simulink model "DFADAS2_SenFus_v1_201204RC_training_210115"  (R2018b)
settings: Solver=FixedStepDiscrete  StartTime=0.0  StopTime=inf  FixedStep=0.002  RelTol=1e-3  EnableMultiTasking=on
PreLoadFcn:
  | RTWConfigurationCB('preloadfcn', bdroot);
libraries: canmsglib x108, simulink x48, canfdmsglib x12
(part 18 of 28)

== system DFADAS2_SenFus_v1_201204RC_training_210115/Signal Input (Input)/Signal Input (50ms) (Input50)/Cmr/CmrInfo/R0 Information (R0Info)/CAN Diagnosis (CANDia)/RollingCounter Diagnosis (RllCntDia) ==
  note: RollingCounter Error Flag Discription:
      | 1 : Fault
      | 0 : Normal
  RllCntChk_ctRollingCounter : Inport
  Add : Sum  Inputs=+-
  Add1 : Sum  Inputs=+-
  Constant : Constant  OutDataTypeStr=single  SampleTime=-1
  Constant1 : Constant  Value=0  OutDataTypeStr=single  SampleTime=-1
  Constant2 : Constant  Value=-1  OutDataTypeStr=single  SampleTime=-1
  Constant3 : Constant  OutDataTypeStr=single  SampleTime=-1
  Data Type Conversion : DataTypeConversion  OutDataTypeStr=single
  Switch : Switch  Criteria=u2 ~= 0
  Switch1 : Switch  Threshold=14.5
  Unit Delay : UnitDelay  SampleTime=-1
  RllCntChk_efErrorFlag : Outport
  wires:
  Switch/1 -> RllCntChk_efErrorFlag/1
  Constant2/1 -> Switch1/1
  Switch1/1 -> Add/2
  Unit Delay/1 -> Switch1/3, Switch1/2
  Data Type Conversion/1 -> Unit Delay/1, Add/1
  Add1/1 -> Switch/2
  Constant3/1 -> Switch/1
  Constant1/1 -> Switch/3
  Constant/1 -> Add1/2
  Add/1 -> Add1/1
  RllCntChk_ctRollingCounter/1 -> Data Type Conversion/1

== system DFADAS2_SenFus_v1_201204RC_training_210115/Signal Input (Input)/Signal Input (50ms) (Input50)/Cmr/CmrInfo/R1 Information (R1Info)/CAN Diagnosis (CANDia)/Break State Diagnosis (BreStDia) ==
  note: Error Flag Discription:
      | 0 : Normal
      | 1 : Fault
  BreStDia_tiCANRxSmplT : Inport
  BreStDia_tiTLim : Inport  Port=2
  BreStDia_cfCANRxNewFlg : Inport  Port=3
  Add : Sum
  Add1 : Sum  Inputs=+-
  Constant : Constant  SampleTime=-1
  Constant1 : Constant  Value=0  SampleTime=-1
  Constant2 : Constant  Value=0  SampleTime=-1
  Constant3 : Constant  SampleTime=-1
  Divide : Product  Inputs=**
  Divide1 : Product  Inputs=/*
  Memory : Memory  InheritSampleTime=on
  Switch : Switch  Criteria=u2 ~= 0
  Switch1 : Switch
  BreStDia_efErrFlg : Outport
  wires:
  Constant1/1 -> Switch/1
  Constant/1 -> Switch/3
  Switch/1 -> Add/1, Divide/2
  Memory/1 -> Add/2
  Divide/1 -> Memory/1
  Add/1 -> Divide/1, Add1/2
  BreStDia_cfCANRxNewFlg/1 -> Switch/2
  BreStDia_tiCANRxSmplT/1 -> Divide1/1
  BreStDia_tiTLim/1 -> Divide1/2
  Add1/1 -> Switch1/2
  Constant2/1 -> Switch1/1
  Constant3/1 -> Switch1/3
  Switch1/1 -> BreStDia_efErrFlg/1
  Divide1/1 -> Add1/1

== system DFADAS2_SenFus_v1_201204RC_training_210115/Signal Input (Input)/Signal Input (50ms) (Input50)/Cmr/CmrInfo/R1 Information (R1Info)/CAN Diagnosis (CANDia)/CAN Frame DTC Generator (CANFrmDTCGtr) ==
  CANFrmDTCGtr_efBreStDiaErrFlg : Inport
  CANFrmDTCGtr_efChkSumDiaErrFlg : Inport  Port=2
  CANFrmDTCGtr_efRllCntDiaErrFlg : Inport  Port=3

== system DFADAS2_SenFus_v1_201204RC_training_210115/Signal Input (Input)/Signal Input (50ms) (Input50)/Cmr/CmrInfo/R1 Information (R1Info)/CAN Diagnosis (CANDia)/CheckSum Diagnosis (ChkSumDia) ==
  ChkSumDia_regCANMsgPrev : Inport
  Bit Check(BChk) : Subsystem  TreatAsAtomicUnit=on
      settings: RTWSystemCode=Nonreusable function
  CAN Message Data Extended (CMsgDaX) : S-Function  FunctionName=CANMsg_DataAcq  SFunctionDeploymentMode=off  EnableBusSupport=off  mask(CANMsg_DataExt){}
      mask help: This block extracts the raw data from the data field of the input CAN frame signal and outputs it as a 1-D array of data type uint8.
      mask Display:
      | color('blue');text(0.98,0.9,'NovSteeds','horizontalAlignment','right');color('black');text(0.5,0.5,'CAN Message\nData Extraction','horizontalAlignment','center');
      | port_label('input',1,'CAN_Msg');
      | port_label('output',1,'RawData');
  ChkSumDia_efErrFlg : Outport
  wires:
  Bit Check(BChk)/1(BChk_efErrFlg) -> ChkSumDia_efErrFlg/1
  ChkSumDia_regCANMsgPrev/1 -> CAN Message Data Extended (CMsgDaX)/1
  CAN Message Data Extended (CMsgDaX)/1 -> Bit Check(BChk)/1(BChk_bRawDa)

== system DFADAS2_SenFus_v1_201204RC_training_210115/Signal Input (Input)/Signal Input (50ms) (Input50)/Cmr/CmrInfo/R1 Information (R1Info)/CAN Diagnosis (CANDia)/RollingCounter Diagnosis (RllCntDia) ==
  note: RollingCounter Error Flag Discription:
      | 1 : Fault
      | 0 : Normal
  RllCntChk_ctRollingCounter : Inport
  Add : Sum  Inputs=+-
  Add1 : Sum  Inputs=+-
  Constant : Constant  OutDataTypeStr=single  SampleTime=-1
  Constant1 : Constant  Value=0  OutDataTypeStr=single  SampleTime=-1
  Constant2 : Constant  Value=-1  OutDataTypeStr=single  SampleTime=-1
  Constant3 : Constant  OutDataTypeStr=single  SampleTime=-1
  Data Type Conversion : DataTypeConversion  OutDataTypeStr=single
  Switch : Switch  Criteria=u2 ~= 0
  Switch1 : Switch  Threshold=14.5
  Unit Delay : UnitDelay  SampleTime=-1
  RllCntChk_efErrorFlag : Outport
  wires:
  RllCntChk_ctRollingCounter/1 -> Data Type Conversion/1
  Add/1 -> Add1/1
  Constant/1 -> Add1/2
  Constant1/1 -> Switch/3
  Constant3/1 -> Switch/1
  Add1/1 -> Switch/2
  Data Type Conversion/1 -> Add/1, Unit Delay/1
  Unit Delay/1 -> Switch1/2, Switch1/3
  Switch1/1 -> Add/2
  Constant2/1 -> Switch1/1
  Switch/1 -> RllCntChk_efErrorFlag/1

== system DFADAS2_SenFus_v1_201204RC_training_210115/Signal Input (Input)/Signal Input (50ms) (Input50)/Front Left Radar(S2) Objects Information (FLRdr)/S0 Data Frame Read/Enabled Subsystem/M0ObjInfo/If Action Subsystem1 ==
  msg : Inport
  "MValueSel " : Inport  Port=2
  obj_trufal : Inport  Port=3
  Action Port : ActionPort  ActionType=then
  Add : Sum
  Add2 : Sum
  MValueSel : Constant  Value=24
  MValueSel2 : Constant  Value=[1:24]
  Product : Product
  Scope1 : Scope
  Selector : Selector  InputPortWidth=240  IndexOptions=Index vector (port)  Indices=[1 3]  OutputSizes=1
  Selector1 : Selector  InputPortWidth=240  IndexOptions=Index vector (port)  Indices=[1 3]  OutputSizes=1
  M00ObjInfo : Outport
  M01ObjInfo : Outport  Port=2
  wires:
  Product/1 -> M01ObjInfo/1
  obj_trufal/1 -> Scope1/1, Product/2
  Selector1/1 -> Product/1
  Selector/1 -> M00ObjInfo/1
  "MValueSel "/1 -> Add2/1
  MValueSel2/1 -> Add2/2
  Add2/1 -> Add/1, Selector/2
  MValueSel/1 -> Add/2
  Add/1 -> Selector1/2
  msg/1 -> Selector1/1, Selector/1

== system DFADAS2_SenFus_v1_201204RC_training_210115/Signal Input (Input)/Signal Input (50ms) (Input50)/Front Left Radar(S2) Objects Information (FLRdr)/S0 Data Frame Read/Enabled Subsystem/M0ObjInfo/If Action Subsystem2 ==
  Action Port : ActionPort  ActionType=elseif
  Constant : Constant  Value=[0 0 0 0 0 0 0 0 0 0 0 0 0 0 0 0 0 0 0 0 0 0 0 0]
  Constant1 : Constant  Value=[0 0 0 0 0 0 0 0 0 0 0 0 0 0 0 0 0 0 0 0 0 0 0 0]
  ZeroObjInfo0 : Outport
  ZeroObjInfo1 : Outport  Port=2
  wires:
  Constant1/1 -> ZeroObjInfo1/1
  Constant/1 -> ZeroObjInfo0/1

== system DFADAS2_SenFus_v1_201204RC_training_210115/Signal Input (Input)/Signal Input (50ms) (Input50)/Front Left Radar(S2) Objects Information (FLRdr)/S0 Data Frame Read/Enabled Subsystem/M0ObjInfo/Subsystem1 ==
  const : Inport
  RemainderCnt : Inport  Port=2
  In : Inport  Port=3
  If : If  IfExpression=u1 >=0
  If Action Subsystem : Subsystem  TreatAsAtomicUnit=on
  If Action Subsystem1 : Subsystem  TreatAsAtomicUnit=on
  Merge : Merge
  Out : Outport
  wires:
  In/1 -> If Action Subsystem1/1(In1)
  const/1 -> If/1
  If/1 -> If Action Subsystem/Action
  If Action Subsystem1/1(Out1) -> Merge/2
  If/2 -> If Action Subsystem1/Action
  Merge/1 -> Out/1
  If Action Subsystem/1(Out1) -> Merge/1

== system DFADAS2_SenFus_v1_201204RC_training_210115/Signal Input (Input)/Signal Input (50ms) (Input50)/Front Left Radar(S2) Objects Information (FLRdr)/S0 Data Frame Read/Enabled Subsystem/M1ObjInfo1/If Action Subsystem1 ==
  msg : Inport
  "MValueSel " : Inport  Port=2
  "0bj_d4 " : Inport  Port=3
  Action Port : ActionPort  ActionType=then
  Add : Sum
  Add2 : Sum
  Gain : Gain  Gain=48
  MValueSel : Constant  Value=24
  MValueSel2 : Constant  Value=[1:24]
  Product : Product
  Scope3 : Scope
  Selector : Selector  InputPortWidth=240  IndexOptions=Index vector (port)  Indices=[1 3]  OutputSizes=1
  Selector1 : Selector  InputPortWidth=240  IndexOptions=Index vector (port)  Indices=[1 3]  OutputSizes=1
  M10ObjInfo : Outport
  M11ObjInfo : Outport  Port=2
  wires:
  Selector/1 -> M10ObjInfo/1
  Product/1 -> M11ObjInfo/1
  "0bj_d4 "/1 -> Scope3/1, Product/2
  "MValueSel "/1 -> Gain/1
  Gain/1 -> Add2/1
  msg/1 -> Selector1/1, Selector/1
  Add/1 -> Selector1/2
  MValueSel/1 -> Add/2
  Add2/1 -> Selector/2, Add/1
  MValueSel2/1 -> Add2/2
  Selector1/1 -> Product/1

== system DFADAS2_SenFus_v1_201204RC_training_210115/Signal Input (Input)/Signal Input (50ms) (Input50)/Front Left Radar(S2) Objects Information (FLRdr)/S0 Data Frame Read/Enabled Subsystem/M1ObjInfo1/If Action Subsystem2 ==
  Action Port : ActionPort  ActionType=elseif
  Constant : Constant  Value=[0 0 0 0 0 0 0 0 0 0 0 0 0 0 0 0 0 0 0 0 0 0 0 0]
  Constant1 : Constant  Value=[0 0 0 0 0 0 0 0 0 0 0 0 0 0 0 0 0 0 0 0 0 0 0 0]
  ZeroObjInfo0 : Outport
  ZeroObjInfo1 : Outport  Port=2
  wires:
  Constant/1 -> ZeroObjInfo0/1
  Constant1/1 -> ZeroObjInfo1/1

== system DFADAS2_SenFus_v1_201204RC_training_210115/Signal Input (Input)/Signal Input (50ms) (Input50)/Front Left Radar(S2) Objects Information (FLRdr)/S0 Data Frame Read/Enabled Subsystem/M1ObjInfo1/Subsystem1 ==
  const : Inport
  RemainderCnt : Inport  Port=2
  In : Inport  Port=3
  If : If  IfExpression=u1 >=0
  If Action Subsystem : Subsystem  TreatAsAtomicUnit=on
  If Action Subsystem1 : Subsystem  TreatAsAtomicUnit=on
  Merge : Merge
  Out : Outport
  wires:
  In/1 -> If Action Subsystem1/1(In1)
  const/1 -> If/1
  If/1 -> If Action Subsystem/Action
  If Action Subsystem1/1(Out1) -> Merge/2
  If/2 -> If Action Subsystem1/Action
  Merge/1 -> Out/1
  If Action Subsystem/1(Out1) -> Merge/1

== system DFADAS2_SenFus_v1_201204RC_training_210115/Signal Input (Input)/Signal Input (50ms) (Input50)/Front Left Radar(S2) Objects Information (FLRdr)/S0 Data Frame Read/Enabled Subsystem/M2ObjInfo/If Action Subsystem1 ==
  msg : Inport
  "MValueSel " : Inport  Port=2
  "obj_count_trorfa " : Inport  Port=3
  Action Port : ActionPort  ActionType=then
  Add : Sum
  Add2 : Sum
  Gain : Gain  Gain=48
  MValueSel : Constant  Value=24
  MValueSel2 : Constant  Value=[1:24]
  Product : Product
  Scope3 : Scope
  Selector : Selector  InputPortWidth=240  IndexOptions=Index vector (port)  Indices=[1 3]  OutputSizes=1
  Selector1 : Selector  InputPortWidth=240  IndexOptions=Index vector (port)  Indices=[1 3]  OutputSizes=1
  M20ObjInfo : Outport
  M21ObjInfo : Outport  Port=2
  wires:
  Product/1 -> M21ObjInfo/1
  "obj_count_trorfa "/1 -> Scope3/1, Product/2
  Selector1/1 -> Product/1
  Selector/1 -> M20ObjInfo/1
  MValueSel2/1 -> Add2/2
  Add2/1 -> Add/1, Selector/2
  MValueSel/1 -> Add/2
  Add/1 -> Selector1/2
  msg/1 -> Selector/1, Selector1/1
  Gain/1 -> Add2/1
  "MValueSel "/1 -> Gain/1

== system DFADAS2_SenFus_v1_201204RC_training_210115/Signal Input (Input)/Signal Input (50ms) (Input50)/Front Left Radar(S2) Objects Information (FLRdr)/S0 Data Frame Read/Enabled Subsystem/M2ObjInfo/If Action Subsystem2 ==
  Action Port : ActionPort  ActionType=elseif
  Constant : Constant  Value=[0 0 0 0 0 0 0 0 0 0 0 0 0 0 0 0 0 0 0 0 0 0 0 0]
  Constant1 : Constant  Value=[0 0 0 0 0 0 0 0 0 0 0 0 0 0 0 0 0 0 0 0 0 0 0 0]
  ZeroObjInfo0 : Outport
  ZeroObjInfo1 : Outport  Port=2
  wires:
  Constant1/1 -> ZeroObjInfo1/1
  Constant/1 -> ZeroObjInfo0/1

== system DFADAS2_SenFus_v1_201204RC_training_210115/Signal Input (Input)/Signal Input (50ms) (Input50)/Front Left Radar(S2) Objects Information (FLRdr)/S0 Data Frame Read/Enabled Subsystem/M2ObjInfo/Subsystem1 ==
  const : Inport
  RemainderCnt : Inport  Port=2
  In : Inport  Port=3
  If : If  IfExpression=u1 >=0
  If Action Subsystem : Subsystem  TreatAsAtomicUnit=on
  If Action Subsystem1 : Subsystem  TreatAsAtomicUnit=on
  Merge : Merge
  Out : Outport
  wires:
  In/1 -> If Action Subsystem1/1(In1)
  const/1 -> If/1
  If/1 -> If Action Subsystem/Action
  If Action Subsystem1/1(Out1) -> Merge/2
  If/2 -> If Action Subsystem1/Action
  Merge/1 -> Out/1
  If Action Subsystem/1(Out1) -> Merge/1

== system DFADAS2_SenFus_v1_201204RC_training_210115/Signal Input (Input)/Signal Input (50ms) (Input50)/Front Left Radar(S2) Objects Information (FLRdr)/S0 Data Frame Read/Enabled Subsystem/M3ObjInfo/If Action Subsystem1 ==
  msg : Inport
  "MValueSel " : Inport  Port=2
  obj_num : Inport  Port=3
  Action Port : ActionPort  ActionType=then
  Add : Sum
  Add2 : Sum
  Gain : Gain  Gain=48
  MValueSel : Constant  Value=24
  MValueSel2 : Constant  Value=[1:24]
  Product : Product
  Scope3 : Scope
  Selector : Selector  InputPortWidth=240  IndexOptions=Index vector (port)  Indices=[1 3]  OutputSizes=1
  Selector1 : Selector  InputPortWidth=240  IndexOptions=Index vector (port)  Indices=[1 3]  OutputSizes=1
  M30ObjInfo : Outport
  M31ObjInfo : Outport  Port=2
  wires:
  Product/1 -> M31ObjInfo/1
  obj_num/1 -> Scope3/1, Product/2
  Selector1/1 -> Product/1
  "MValueSel "/1 -> Gain/1
  Gain/1 -> Add2/1
  msg/1 -> Selector1/1, Selector/1
  Add/1 -> Selector1/2
  MValueSel/1 -> Add/2
  Add2/1 -> Selector/2, Add/1
  MValueSel2/1 -> Add2/2
  Selector/1 -> M30ObjInfo/1

== system DFADAS2_SenFus_v1_201204RC_training_210115/Signal Input (Input)/Signal Input (50ms) (Input50)/Front Left Radar(S2) Objects Information (FLRdr)/S0 Data Frame Read/Enabled Subsystem/M3ObjInfo/If Action Subsystem2 ==
  Action Port : ActionPort  ActionType=elseif
  Constant : Constant  Value=[0 0 0 0 0 0 0 0 0 0 0 0 0 0 0 0 0 0 0 0 0 0 0 0]
  Constant1 : Constant  Value=[0 0 0 0 0 0 0 0 0 0 0 0 0 0 0 0 0 0 0 0 0 0 0 0]
  ZeroObjInfo0 : Outport
  ZeroObjInfo1 : Outport  Port=2
  wires:
  Constant/1 -> ZeroObjInfo0/1
  Constant1/1 -> ZeroObjInfo1/1

== system DFADAS2_SenFus_v1_201204RC_training_210115/Signal Input (Input)/Signal Input (50ms) (Input50)/Front Left Radar(S2) Objects Information (FLRdr)/S0 Data Frame Read/Enabled Subsystem/M3ObjInfo/Subsystem1 ==
  const : Inport
  RemainderCnt : Inport  Port=2
  In : Inport  Port=3
  If : If  IfExpression=u1 >=0
  If Action Subsystem : Subsystem  TreatAsAtomicUnit=on
  If Action Subsystem1 : Subsystem  TreatAsAtomicUnit=on
  Merge : Merge
  Out : Outport
  wires:
  In/1 -> If Action Subsystem1/1(In1)
  const/1 -> If/1
  If/1 -> If Action Subsystem/Action
  If Action Subsystem1/1(Out1) -> Merge/2
  If/2 -> If Action Subsystem1/Action
  Merge/1 -> Out/1
  If Action Subsystem/1(Out1) -> Merge/1

== system DFADAS2_SenFus_v1_201204RC_training_210115/Signal Input (Input)/Signal Input (50ms) (Input50)/Front Left Radar(S2) Objects Information (FLRdr)/S0 Data Frame Read/Enabled Subsystem/M4ObjInfo1/If Action Subsystem1 ==
  msg : Inport
  "MValueSel " : Inport  Port=2
  "obj_num " : Inport  Port=3
  Action Port : ActionPort  ActionType=then
  Add : Sum
  Add2 : Sum
  Gain : Gain  Gain=48
  MValueSel : Constant  Value=24
  MValueSel2 : Constant  Value=[1:24]
  Product : Product
  Scope3 : Scope
  Selector : Selector  InputPortWidth=240  IndexOptions=Index vector (port)  Indices=[1 3]  OutputSizes=1
  Selector1 : Selector  InputPortWidth=240  IndexOptions=Index vector (port)  Indices=[1 3]  OutputSizes=1
  M40ObjInfo : Outport
  M41ObjInfo : Outport  Port=2
  wires:
  Product/1 -> M41ObjInfo/1
  "obj_num "/1 -> Scope3/1, Product/2
  Selector1/1 -> Product/1
  Selector/1 -> M40ObjInfo/1
  MValueSel2/1 -> Add2/2
  Add2/1 -> Add/1, Selector/2
  MValueSel/1 -> Add/2
  Add/1 -> Selector1/2
  msg/1 -> Selector/1, Selector1/1
  Gain/1 -> Add2/1
  "MValueSel "/1 -> Gain/1

== system DFADAS2_SenFus_v1_201204RC_training_210115/Signal Input (Input)/Signal Input (50ms) (Input50)/Front Left Radar(S2) Objects Information (FLRdr)/S0 Data Frame Read/Enabled Subsystem/M4ObjInfo1/If Action Subsystem2 ==
  Action Port : ActionPort  ActionType=elseif
  Constant : Constant  Value=[0 0 0 0 0 0 0 0 0 0 0 0 0 0 0 0 0 0 0 0 0 0 0 0]
  Constant1 : Constant  Value=[0 0 0 0 0 0 0 0 0 0 0 0 0 0 0 0 0 0 0 0 0 0 0 0]
  ZeroObjInfo0 : Outport
  ZeroObjInfo1 : Outport  Port=2
  wires:
  Constant1/1 -> ZeroObjInfo1/1
  Constant/1 -> ZeroObjInfo0/1

== system DFADAS2_SenFus_v1_201204RC_training_210115/Signal Input (Input)/Signal Input (50ms) (Input50)/Front Left Radar(S2) Objects Information (FLRdr)/S0 Data Frame Read/Enabled Subsystem/M4ObjInfo1/Subsystem1 ==
  const : Inport
  RemainderCnt : Inport  Port=2
  In : Inport  Port=3
  If : If  IfExpression=u1 >=0
  If Action Subsystem : Subsystem  TreatAsAtomicUnit=on
  If Action Subsystem1 : Subsystem  TreatAsAtomicUnit=on
  Merge : Merge
  Out : Outport
  wires:
  In/1 -> If Action Subsystem1/1(In1)
  const/1 -> If/1
  If/1 -> If Action Subsystem/Action
  If Action Subsystem1/1(Out1) -> Merge/2
  If/2 -> If Action Subsystem1/Action
  Merge/1 -> Out/1
  If Action Subsystem/1(Out1) -> Merge/1

== system DFADAS2_SenFus_v1_201204RC_training_210115/Signal Input (Input)/Signal Input (50ms) (Input50)/Front Left Radar(S2) Objects Information (FLRdr)/S0 Data Frame Read/Enabled Subsystem/Unpack/If Action Subsystem ==
  msg : Inport
  Action Port : ActionPort  ActionType=then
  Unpack : Subsystem
  FLRdrObjInfo : Outport
  MValue : Outport  Port=2
  wires:
  Unpack/2(MValue) -> MValue/1
  msg/1 -> Unpack/1(msg)
  Unpack/1(FLRdrObjInfo) -> FLRdrObjInfo/1

== system DFADAS2_SenFus_v1_201204RC_training_210115/Signal Input (Input)/Signal Input (50ms) (Input50)/Front Left Radar(S2) Objects Information (FLRdr)/S0 Data Frame Read/Enabled Subsystem/Unpack/If Action Subsystem1 ==
  Action Port : ActionPort  ActionType=elseif
  Constant : Constant  Value=99
  DflMValue : Outport
  wires:
  Constant/1 -> DflMValue/1

== system DFADAS2_SenFus_v1_201204RC_training_210115/Signal Input (Input)/Signal Input (50ms) (Input50)/Front Right Radar(S3) Objects Information (FRRdr)/S0 Data Frame Read/Enabled Subsystem/M0ObjInfo/If Action Subsystem1 ==
  msg : Inport
  "MValueSel " : Inport  Port=2
  obj_trufal : Inport  Port=3
  Action Port : ActionPort  ActionType=then
  Add : Sum
  Add2 : Sum
  MValueSel : Constant  Value=24
  MValueSel2 : Constant  Value=[1:24]
  Product : Product
  Scope1 : Scope
  Selector : Selector  InputPortWidth=240  IndexOptions=Index vector (port)  Indices=[1 3]  OutputSizes=1
  Selector1 : Selector  InputPortWidth=240  IndexOptions=Index vector (port)  Indices=[1 3]  OutputSizes=1
  M00ObjInfo : Outport
  M01ObjInfo : Outport  Port=2
  wires:
  msg/1 -> Selector/1, Selector1/1
  Add/1 -> Selector1/2
  MValueSel/1 -> Add/2
  Add2/1 -> Selector/2, Add/1
  MValueSel2/1 -> Add2/2
  "MValueSel "/1 -> Add2/1
  Selector/1 -> M00ObjInfo/1
  Selector1/1 -> Product/1
  obj_trufal/1 -> Product/2, Scope1/1
  Product/1 -> M01ObjInfo/1

== system DFADAS2_SenFus_v1_201204RC_training_210115/Signal Input (Input)/Signal Input (50ms) (Input50)/Front Right Radar(S3) Objects Information (FRRdr)/S0 Data Frame Read/Enabled Subsystem/M0ObjInfo/If Action Subsystem2 ==
  Action Port : ActionPort  ActionType=elseif
  Constant : Constant  Value=[0 0 0 0 0 0 0 0 0 0 0 0 0 0 0 0 0 0 0 0 0 0 0 0]
  Constant1 : Constant  Value=[0 0 0 0 0 0 0 0 0 0 0 0 0 0 0 0 0 0 0 0 0 0 0 0]
  ZeroObjInfo0 : Outport
  ZeroObjInfo1 : Outport  Port=2
  wires:
  Constant/1 -> ZeroObjInfo0/1
  Constant1/1 -> ZeroObjInfo1/1

== system DFADAS2_SenFus_v1_201204RC_training_210115/Signal Input (Input)/Signal Input (50ms) (Input50)/Front Right Radar(S3) Objects Information (FRRdr)/S0 Data Frame Read/Enabled Subsystem/M0ObjInfo/Subsystem1 ==
  const : Inport
  RemainderCnt : Inport  Port=2
  In : Inport  Port=3
  If : If  IfExpression=u1 >=0
  If Action Subsystem : Subsystem  TreatAsAtomicUnit=on
  If Action Subsystem1 : Subsystem  TreatAsAtomicUnit=on
  Merge : Merge
  Out : Outport
  wires:
  If Action Subsystem/1(Out1) -> Merge/1
  Merge/1 -> Out/1
  If/2 -> If Action Subsystem1/Action
  If Action Subsystem1/1(Out1) -> Merge/2
  If/1 -> If Action Subsystem/Action
  const/1 -> If/1
  In/1 -> If Action Subsystem1/1(In1)

== system DFADAS2_SenFus_v1_201204RC_training_210115/Signal Input (Input)/Signal Input (50ms) (Input50)/Front Right Radar(S3) Objects Information (FRRdr)/S0 Data Frame Read/Enabled Subsystem/M1ObjInfo1/If Action Subsystem1 ==
  msg : Inport
  "MValueSel " : Inport  Port=2
  "0bj_d4 " : Inport  Port=3
  Action Port : ActionPort  ActionType=then
  Add : Sum
  Add2 : Sum
  Gain : Gain  Gain=48
  MValueSel : Constant  Value=24
  MValueSel2 : Constant  Value=[1:24]
  Product : Product
  Scope3 : Scope
  Selector : Selector  InputPortWidth=240  IndexOptions=Index vector (port)  Indices=[1 3]  OutputSizes=1
  Selector1 : Selector  InputPortWidth=240  IndexOptions=Index vector (port)  Indices=[1 3]  OutputSizes=1
  M10ObjInfo : Outport
  M11ObjInfo : Outport  Port=2
  wires:
  Selector1/1 -> Product/1
  MValueSel2/1 -> Add2/2
  Add2/1 -> Add/1, Selector/2
  MValueSel/1 -> Add/2
  Add/1 -> Selector1/2
  msg/1 -> Selector/1, Selector1/1
  Gain/1 -> Add2/1
  "MValueSel "/1 -> Gain/1
  "0bj_d4 "/1 -> Product/2, Scope3/1
  Product/1 -> M11ObjInfo/1
  Selector/1 -> M10ObjInfo/1

== system DFADAS2_SenFus_v1_201204RC_training_210115/Signal Input (Input)/Signal Input (50ms) (Input50)/Front Right Radar(S3) Objects Information (FRRdr)/S0 Data Frame Read/Enabled Subsystem/M1ObjInfo1/If Action Subsystem2 ==
  Action Port : ActionPort  ActionType=elseif
  Constant : Constant  Value=[0 0 0 0 0 0 0 0 0 0 0 0 0 0 0 0 0 0 0 0 0 0 0 0]
  Constant1 : Constant  Value=[0 0 0 0 0 0 0 0 0 0 0 0 0 0 0 0 0 0 0 0 0 0 0 0]
  ZeroObjInfo0 : Outport
  ZeroObjInfo1 : Outport  Port=2
  wires:
  Constant1/1 -> ZeroObjInfo1/1
  Constant/1 -> ZeroObjInfo0/1

== system DFADAS2_SenFus_v1_201204RC_training_210115/Signal Input (Input)/Signal Input (50ms) (Input50)/Front Right Radar(S3) Objects Information (FRRdr)/S0 Data Frame Read/Enabled Subsystem/M1ObjInfo1/Subsystem1 ==
  const : Inport
  RemainderCnt : Inport  Port=2
  In : Inport  Port=3
  If : If  IfExpression=u1 >=0
  If Action Subsystem : Subsystem  TreatAsAtomicUnit=on
  If Action Subsystem1 : Subsystem  TreatAsAtomicUnit=on
  Merge : Merge
  Out : Outport
  wires:
  If Action Subsystem/1(Out1) -> Merge/1
  Merge/1 -> Out/1
  If/2 -> If Action Subsystem1/Action
  If Action Subsystem1/1(Out1) -> Merge/2
  If/1 -> If Action Subsystem/Action
  const/1 -> If/1
  In/1 -> If Action Subsystem1/1(In1)

== system DFADAS2_SenFus_v1_201204RC_training_210115/Signal Input (Input)/Signal Input (50ms) (Input50)/Front Right Radar(S3) Objects Information (FRRdr)/S0 Data Frame Read/Enabled Subsystem/M2ObjInfo/If Action Subsystem1 ==
  msg : Inport
  "MValueSel " : Inport  Port=2
  "obj_count_trorfa " : Inport  Port=3
  Action Port : ActionPort  ActionType=then
  Add : Sum
  Add2 : Sum
  Gain : Gain  Gain=48
  MValueSel : Constant  Value=24
  MValueSel2 : Constant  Value=[1:24]
  Product : Product
  Scope3 : Scope
  Selector : Selector  InputPortWidth=240  IndexOptions=Index vector (port)  Indices=[1 3]  OutputSizes=1
  Selector1 : Selector  InputPortWidth=240  IndexOptions=Index vector (port)  Indices=[1 3]  OutputSizes=1
  M20ObjInfo : Outport
  M21ObjInfo : Outport  Port=2
  wires:
  "MValueSel "/1 -> Gain/1
  Gain/1 -> Add2/1
  msg/1 -> Selector1/1, Selector/1
  Add/1 -> Selector1/2
  MValueSel/1 -> Add/2
  Add2/1 -> Selector/2, Add/1
  MValueSel2/1 -> Add2/2
  Selector/1 -> M20ObjInfo/1
  Selector1/1 -> Product/1
  "obj_count_trorfa "/1 -> Product/2, Scope3/1
  Product/1 -> M21ObjInfo/1

== system DFADAS2_SenFus_v1_201204RC_training_210115/Signal Input (Input)/Signal Input (50ms) (Input50)/Front Right Radar(S3) Objects Information (FRRdr)/S0 Data Frame Read/Enabled Subsystem/M2ObjInfo/If Action Subsystem2 ==
  Action Port : ActionPort  ActionType=elseif
  Constant : Constant  Value=[0 0 0 0 0 0 0 0 0 0 0 0 0 0 0 0 0 0 0 0 0 0 0 0]
  Constant1 : Constant  Value=[0 0 0 0 0 0 0 0 0 0 0 0 0 0 0 0 0 0 0 0 0 0 0 0]
  ZeroObjInfo0 : Outport
  ZeroObjInfo1 : Outport  Port=2
  wires:
  Constant/1 -> ZeroObjInfo0/1
  Constant1/1 -> ZeroObjInfo1/1

== system DFADAS2_SenFus_v1_201204RC_training_210115/Signal Input (Input)/Signal Input (50ms) (Input50)/Front Right Radar(S3) Objects Information (FRRdr)/S0 Data Frame Read/Enabled Subsystem/M2ObjInfo/Subsystem1 ==
  const : Inport
  RemainderCnt : Inport  Port=2
  In : Inport  Port=3
  If : If  IfExpression=u1 >=0
  If Action Subsystem : Subsystem  TreatAsAtomicUnit=on
  If Action Subsystem1 : Subsystem  TreatAsAtomicUnit=on
  Merge : Merge
  Out : Outport
  wires:
  If Action Subsystem/1(Out1) -> Merge/1
  Merge/1 -> Out/1
  If/2 -> If Action Subsystem1/Action
  If Action Subsystem1/1(Out1) -> Merge/2
  If/1 -> If Action Subsystem/Action
  const/1 -> If/1
  In/1 -> If Action Subsystem1/1(In1)

== system DFADAS2_SenFus_v1_201204RC_training_210115/Signal Input (Input)/Signal Input (50ms) (Input50)/Front Right Radar(S3) Objects Information (FRRdr)/S0 Data Frame Read/Enabled Subsystem/M3ObjInfo/If Action Subsystem1 ==
  msg : Inport
  "MValueSel " : Inport  Port=2
  obj_num : Inport  Port=3
  Action Port : ActionPort  ActionType=then
  Add : Sum
  Add2 : Sum
  Gain : Gain  Gain=48
  MValueSel : Constant  Value=24
  MValueSel2 : Constant  Value=[1:24]
  Product : Product
  Scope3 : Scope
  Selector : Selector  InputPortWidth=240  IndexOptions=Index vector (port)  Indices=[1 3]  OutputSizes=1
  Selector1 : Selector  InputPortWidth=240  IndexOptions=Index vector (port)  Indices=[1 3]  OutputSizes=1
  M30ObjInfo : Outport
  M31ObjInfo : Outport  Port=2
  wires:
  Selector/1 -> M30ObjInfo/1
  MValueSel2/1 -> Add2/2
  Add2/1 -> Add/1, Selector/2
  MValueSel/1 -> Add/2
  Add/1 -> Selector1/2
  msg/1 -> Selector/1, Selector1/1
  Gain/1 -> Add2/1
  "MValueSel "/1 -> Gain/1
  Selector1/1 -> Product/1
  obj_num/1 -> Product/2, Scope3/1
  Product/1 -> M31ObjInfo/1

== system DFADAS2_SenFus_v1_201204RC_training_210115/Signal Input (Input)/Signal Input (50ms) (Input50)/Front Right Radar(S3) Objects Information (FRRdr)/S0 Data Frame Read/Enabled Subsystem/M3ObjInfo/If Action Subsystem2 ==
  Action Port : ActionPort  ActionType=elseif
  Constant : Constant  Value=[0 0 0 0 0 0 0 0 0 0 0 0 0 0 0 0 0 0 0 0 0 0 0 0]
  Constant1 : Constant  Value=[0 0 0 0 0 0 0 0 0 0 0 0 0 0 0 0 0 0 0 0 0 0 0 0]
  ZeroObjInfo0 : Outport
  ZeroObjInfo1 : Outport  Port=2
  wires:
  Constant1/1 -> ZeroObjInfo1/1
  Constant/1 -> ZeroObjInfo0/1

== system DFADAS2_SenFus_v1_201204RC_training_210115/Signal Input (Input)/Signal Input (50ms) (Input50)/Front Right Radar(S3) Objects Information (FRRdr)/S0 Data Frame Read/Enabled Subsystem/M3ObjInfo/Subsystem1 ==
  const : Inport
  RemainderCnt : Inport  Port=2
  In : Inport  Port=3
  If : If  IfExpression=u1 >=0
  If Action Subsystem : Subsystem  TreatAsAtomicUnit=on
  If Action Subsystem1 : Subsystem  TreatAsAtomicUnit=on
  Merge : Merge
  Out : Outport
  wires:
  If Action Subsystem/1(Out1) -> Merge/1
  Merge/1 -> Out/1
  If/2 -> If Action Subsystem1/Action
  If Action Subsystem1/1(Out1) -> Merge/2
  If/1 -> If Action Subsystem/Action
  const/1 -> If/1
  In/1 -> If Action Subsystem1/1(In1)

== system DFADAS2_SenFus_v1_201204RC_training_210115/Signal Input (Input)/Signal Input (50ms) (Input50)/Front Right Radar(S3) Objects Information (FRRdr)/S0 Data Frame Read/Enabled Subsystem/M4ObjInfo1/If Action Subsystem1 ==
  msg : Inport
  "MValueSel " : Inport  Port=2
  "obj_num " : Inport  Port=3
  Action Port : ActionPort  ActionType=then
  Add : Sum
  Add2 : Sum
  Gain : Gain  Gain=48
  MValueSel : Constant  Value=24
  MValueSel2 : Constant  Value=[1:24]
  Product : Product
  Scope3 : Scope
  Selector : Selector  InputPortWidth=240  IndexOptions=Index vector (port)  Indices=[1 3]  OutputSizes=1
  Selector1 : Selector  InputPortWidth=240  IndexOptions=Index vector (port)  Indices=[1 3]  OutputSizes=1
  M40ObjInfo : Outport
  M41ObjInfo : Outport  Port=2
  wires:
  "MValueSel "/1 -> Gain/1
  Gain/1 -> Add2/1
  msg/1 -> Selector1/1, Selector/1
  Add/1 -> Selector1/2
  MValueSel/1 -> Add/2
  Add2/1 -> Selector/2, Add/1
  MValueSel2/1 -> Add2/2
  Selector/1 -> M40ObjInfo/1
  Selector1/1 -> Product/1
  "obj_num "/1 -> Product/2, Scope3/1
  Product/1 -> M41ObjInfo/1

== system DFADAS2_SenFus_v1_201204RC_training_210115/Signal Input (Input)/Signal Input (50ms) (Input50)/Front Right Radar(S3) Objects Information (FRRdr)/S0 Data Frame Read/Enabled Subsystem/M4ObjInfo1/If Action Subsystem2 ==
  Action Port : ActionPort  ActionType=elseif
  Constant : Constant  Value=[0 0 0 0 0 0 0 0 0 0 0 0 0 0 0 0 0 0 0 0 0 0 0 0]
  Constant1 : Constant  Value=[0 0 0 0 0 0 0 0 0 0 0 0 0 0 0 0 0 0 0 0 0 0 0 0]
  ZeroObjInfo0 : Outport
  ZeroObjInfo1 : Outport  Port=2
  wires:
  Constant/1 -> ZeroObjInfo0/1
  Constant1/1 -> ZeroObjInfo1/1

== system DFADAS2_SenFus_v1_201204RC_training_210115/Signal Input (Input)/Signal Input (50ms) (Input50)/Front Right Radar(S3) Objects Information (FRRdr)/S0 Data Frame Read/Enabled Subsystem/M4ObjInfo1/Subsystem1 ==
  const : Inport
  RemainderCnt : Inport  Port=2
  In : Inport  Port=3
  If : If  IfExpression=u1 >=0
  If Action Subsystem : Subsystem  TreatAsAtomicUnit=on
  If Action Subsystem1 : Subsystem  TreatAsAtomicUnit=on
  Merge : Merge
  Out : Outport
  wires:
  If Action Subsystem/1(Out1) -> Merge/1
  Merge/1 -> Out/1
  If/2 -> If Action Subsystem1/Action
  If Action Subsystem1/1(Out1) -> Merge/2
  If/1 -> If Action Subsystem/Action
  const/1 -> If/1
  In/1 -> If Action Subsystem1/1(In1)

== system DFADAS2_SenFus_v1_201204RC_training_210115/Signal Input (Input)/Signal Input (50ms) (Input50)/Front Right Radar(S3) Objects Information (FRRdr)/S0 Data Frame Read/Enabled Subsystem/Unpack/If Action Subsystem ==
  msg : Inport
  Action Port : ActionPort  ActionType=then
  Unpack : Subsystem
  FRRdrObjInfo : Outport
  MValue : Outport  Port=2
  wires:
  Unpack/2(MValue) -> MValue/1
  msg/1 -> Unpack/1(msg)
  Unpack/1(FRRdrObjInfo) -> FRRdrObjInfo/1

== system DFADAS2_SenFus_v1_201204RC_training_210115/Signal Input (Input)/Signal Input (50ms) (Input50)/Front Right Radar(S3) Objects Information (FRRdr)/S0 Data Frame Read/Enabled Subsystem/Unpack/If Action Subsystem1 ==
  Action Port : ActionPort  ActionType=elseif
  Constant : Constant  Value=99
  DflMValue : Outport
  wires:
  Constant/1 -> DflMValue/1

== system DFADAS2_SenFus_v1_201204RC_training_210115/Signal Input (Input)/Signal Input (50ms) (Input50)/Rear Left Radar(S0) Objects Information (RLRdr)/S0 Data Frame Read/Enabled Subsystem/M0ObjInfo/If Action Subsystem1 ==
  msg : Inport
  "MValueSel " : Inport  Port=2
  obj_trufal : Inport  Port=3
  Action Port : ActionPort  ActionType=then
  Add : Sum
  Add2 : Sum
  MValueSel : Constant  Value=24
  MValueSel2 : Constant  Value=[1:24]
  Product : Product
  Scope1 : Scope
  Selector : Selector  InputPortWidth=240  IndexOptions=Index vector (port)  Indices=[1 3]  OutputSizes=1
  Selector1 : Selector  InputPortWidth=240  IndexOptions=Index vector (port)  Indices=[1 3]  OutputSizes=1
  M00ObjInfo : Outport
  M01ObjInfo : Outport  Port=2
  wires:
  msg/1 -> Selector/1, Selector1/1
  Add/1 -> Selector1/2
  MValueSel/1 -> Add/2
  Add2/1 -> Selector/2, Add/1
  MValueSel2/1 -> Add2/2
  "MValueSel "/1 -> Add2/1
  Selector/1 -> M00ObjInfo/1
  Selector1/1 -> Product/1
  obj_trufal/1 -> Product/2, Scope1/1
  Product/1 -> M01ObjInfo/1

== system DFADAS2_SenFus_v1_201204RC_training_210115/Signal Input (Input)/Signal Input (50ms) (Input50)/Rear Left Radar(S0) Objects Information (RLRdr)/S0 Data Frame Read/Enabled Subsystem/M0ObjInfo/If Action Subsystem2 ==
  Action Port : ActionPort  ActionType=elseif
  Constant : Constant  Value=[0 0 0 0 0 0 0 0 0 0 0 0 0 0 0 0 0 0 0 0 0 0 0 0]
  Constant1 : Constant  Value=[0 0 0 0 0 0 0 0 0 0 0 0 0 0 0 0 0 0 0 0 0 0 0 0]
  ZeroObjInfo0 : Outport
  ZeroObjInfo1 : Outport  Port=2
  wires:
  Constant/1 -> ZeroObjInfo0/1
  Constant1/1 -> ZeroObjInfo1/1

== system DFADAS2_SenFus_v1_201204RC_training_210115/Signal Input (Input)/Signal Input (50ms) (Input50)/Rear Left Radar(S0) Objects Information (RLRdr)/S0 Data Frame Read/Enabled Subsystem/M0ObjInfo/Subsystem1 ==
  const : Inport
  RemainderCnt : Inport  Port=2
  In : Inport  Port=3
  If : If  IfExpression=u1 >=0
  If Action Subsystem : Subsystem  TreatAsAtomicUnit=on
  If Action Subsystem1 : Subsystem  TreatAsAtomicUnit=on
  Merge : Merge
  Out : Outport
  wires:
  If Action Subsystem/1(Out1) -> Merge/1
  Merge/1 -> Out/1
  If/2 -> If Action Subsystem1/Action
  If Action Subsystem1/1(Out1) -> Merge/2
  If/1 -> If Action Subsystem/Action
  const/1 -> If/1
  In/1 -> If Action Subsystem1/1(In1)

== system DFADAS2_SenFus_v1_201204RC_training_210115/Signal Input (Input)/Signal Input (50ms) (Input50)/Rear Left Radar(S0) Objects Information (RLRdr)/S0 Data Frame Read/Enabled Subsystem/M1ObjInfo1/If Action Subsystem1 ==
  msg : Inport
  "MValueSel " : Inport  Port=2
  "0bj_d4 " : Inport  Port=3
  Action Port : ActionPort  ActionType=then
  Add : Sum
  Add2 : Sum
  Gain : Gain  Gain=48
  MValueSel : Constant  Value=24
  MValueSel2 : Constant  Value=[1:24]
  Product : Product
  Scope3 : Scope
  Selector : Selector  InputPortWidth=240  IndexOptions=Index vector (port)  Indices=[1 3]  OutputSizes=1
  Selector1 : Selector  InputPortWidth=240  IndexOptions=Index vector (port)  Indices=[1 3]  OutputSizes=1
  M10ObjInfo : Outport
  M11ObjInfo : Outport  Port=2
  wires:
  Selector1/1 -> Product/1
  MValueSel2/1 -> Add2/2
  Add2/1 -> Add/1, Selector/2
  MValueSel/1 -> Add/2
  Add/1 -> Selector1/2
  msg/1 -> Selector/1, Selector1/1
  Gain/1 -> Add2/1
  "MValueSel "/1 -> Gain/1
  "0bj_d4 "/1 -> Product/2, Scope3/1
  Product/1 -> M11ObjInfo/1
  Selector/1 -> M10ObjInfo/1

== system DFADAS2_SenFus_v1_201204RC_training_210115/Signal Input (Input)/Signal Input (50ms) (Input50)/Rear Left Radar(S0) Objects Information (RLRdr)/S0 Data Frame Read/Enabled Subsystem/M1ObjInfo1/If Action Subsystem2 ==
  Action Port : ActionPort  ActionType=elseif
  Constant : Constant  Value=[0 0 0 0 0 0 0 0 0 0 0 0 0 0 0 0 0 0 0 0 0 0 0 0]
  Constant1 : Constant  Value=[0 0 0 0 0 0 0 0 0 0 0 0 0 0 0 0 0 0 0 0 0 0 0 0]
  ZeroObjInfo0 : Outport
  ZeroObjInfo1 : Outport  Port=2
  wires:
  Constant1/1 -> ZeroObjInfo1/1
  Constant/1 -> ZeroObjInfo0/1

== system DFADAS2_SenFus_v1_201204RC_training_210115/Signal Input (Input)/Signal Input (50ms) (Input50)/Rear Left Radar(S0) Objects Information (RLRdr)/S0 Data Frame Read/Enabled Subsystem/M1ObjInfo1/Subsystem1 ==
  const : Inport
  RemainderCnt : Inport  Port=2
  In : Inport  Port=3
  If : If  IfExpression=u1 >=0
  If Action Subsystem : Subsystem  TreatAsAtomicUnit=on
  If Action Subsystem1 : Subsystem  TreatAsAtomicUnit=on
  Merge : Merge
  Out : Outport
  wires:
  If Action Subsystem/1(Out1) -> Merge/1
  Merge/1 -> Out/1
  If/2 -> If Action Subsystem1/Action
  If Action Subsystem1/1(Out1) -> Merge/2
  If/1 -> If Action Subsystem/Action
  const/1 -> If/1
  In/1 -> If Action Subsystem1/1(In1)

== system DFADAS2_SenFus_v1_201204RC_training_210115/Signal Input (Input)/Signal Input (50ms) (Input50)/Rear Left Radar(S0) Objects Information (RLRdr)/S0 Data Frame Read/Enabled Subsystem/M2ObjInfo/If Action Subsystem1 ==
  msg : Inport
  "MValueSel " : Inport  Port=2
  "obj_count_trorfa " : Inport  Port=3
  Action Port : ActionPort  ActionType=then
  Add : Sum
  Add2 : Sum
  Gain : Gain  Gain=48
  MValueSel : Constant  Value=24
  MValueSel2 : Constant  Value=[1:24]
  Product : Product
  Scope3 : Scope
  Selector : Selector  InputPortWidth=240  IndexOptions=Index vector (port)  Indices=[1 3]  OutputSizes=1
  Selector1 : Selector  InputPortWidth=240  IndexOptions=Index vector (port)  Indices=[1 3]  OutputSizes=1
  M20ObjInfo : Outport
  M21ObjInfo : Outport  Port=2
  wires:
  "MValueSel "/1 -> Gain/1
  Gain/1 -> Add2/1
  msg/1 -> Selector1/1, Selector/1
  Add/1 -> Selector1/2
  MValueSel/1 -> Add/2
  Add2/1 -> Selector/2, Add/1
  MValueSel2/1 -> Add2/2
  Selector/1 -> M20ObjInfo/1
  Selector1/1 -> Product/1
  "obj_count_trorfa "/1 -> Product/2, Scope3/1
  Product/1 -> M21ObjInfo/1

== system DFADAS2_SenFus_v1_201204RC_training_210115/Signal Input (Input)/Signal Input (50ms) (Input50)/Rear Left Radar(S0) Objects Information (RLRdr)/S0 Data Frame Read/Enabled Subsystem/M2ObjInfo/If Action Subsystem2 ==
  Action Port : ActionPort  ActionType=elseif
  Constant : Constant  Value=[0 0 0 0 0 0 0 0 0 0 0 0 0 0 0 0 0 0 0 0 0 0 0 0]
  Constant1 : Constant  Value=[0 0 0 0 0 0 0 0 0 0 0 0 0 0 0 0 0 0 0 0 0 0 0 0]
  ZeroObjInfo0 : Outport
  ZeroObjInfo1 : Outport  Port=2
  wires:
  Constant/1 -> ZeroObjInfo0/1
  Constant1/1 -> ZeroObjInfo1/1

== system DFADAS2_SenFus_v1_201204RC_training_210115/Signal Input (Input)/Signal Input (50ms) (Input50)/Rear Left Radar(S0) Objects Information (RLRdr)/S0 Data Frame Read/Enabled Subsystem/M2ObjInfo/Subsystem1 ==
  const : Inport
  RemainderCnt : Inport  Port=2
  In : Inport  Port=3
  If : If  IfExpression=u1 >=0
  If Action Subsystem : Subsystem  TreatAsAtomicUnit=on
  If Action Subsystem1 : Subsystem  TreatAsAtomicUnit=on
  Merge : Merge
  Out : Outport
  wires:
  If Action Subsystem/1(Out1) -> Merge/1
  Merge/1 -> Out/1
  If/2 -> If Action Subsystem1/Action
  If Action Subsystem1/1(Out1) -> Merge/2
  If/1 -> If Action Subsystem/Action
  const/1 -> If/1
  In/1 -> If Action Subsystem1/1(In1)

== system DFADAS2_SenFus_v1_201204RC_training_210115/Signal Input (Input)/Signal Input (50ms) (Input50)/Rear Left Radar(S0) Objects Information (RLRdr)/S0 Data Frame Read/Enabled Subsystem/M3ObjInfo/If Action Subsystem1 ==
  msg : Inport
  "MValueSel " : Inport  Port=2
  obj_num : Inport  Port=3
  Action Port : ActionPort  ActionType=then
  Add : Sum
  Add2 : Sum
  Gain : Gain  Gain=48
  MValueSel : Constant  Value=24
  MValueSel2 : Constant  Value=[1:24]
  Product : Product
  Scope3 : Scope
  Selector : Selector  InputPortWidth=240  IndexOptions=Index vector (port)  Indices=[1 3]  OutputSizes=1
  Selector1 : Selector  InputPortWidth=240  IndexOptions=Index vector (port)  Indices=[1 3]  OutputSizes=1
  M30ObjInfo : Outport
  M31ObjInfo : Outport  Port=2
  wires:
  Selector/1 -> M30ObjInfo/1
  MValueSel2/1 -> Add2/2
  Add2/1 -> Add/1, Selector/2
  MValueSel/1 -> Add/2
  Add/1 -> Selector1/2
  msg/1 -> Selector/1, Selector1/1
  Gain/1 -> Add2/1
  "MValueSel "/1 -> Gain/1
  Selector1/1 -> Product/1
  obj_num/1 -> Product/2, Scope3/1
  Product/1 -> M31ObjInfo/1

== system DFADAS2_SenFus_v1_201204RC_training_210115/Signal Input (Input)/Signal Input (50ms) (Input50)/Rear Left Radar(S0) Objects Information (RLRdr)/S0 Data Frame Read/Enabled Subsystem/M3ObjInfo/If Action Subsystem2 ==
  Action Port : ActionPort  ActionType=elseif
  Constant : Constant  Value=[0 0 0 0 0 0 0 0 0 0 0 0 0 0 0 0 0 0 0 0 0 0 0 0]
  Constant1 : Constant  Value=[0 0 0 0 0 0 0 0 0 0 0 0 0 0 0 0 0 0 0 0 0 0 0 0]
  ZeroObjInfo0 : Outport
  ZeroObjInfo1 : Outport  Port=2
  wires:
  Constant1/1 -> ZeroObjInfo1/1
  Constant/1 -> ZeroObjInfo0/1

== system DFADAS2_SenFus_v1_201204RC_training_210115/Signal Input (Input)/Signal Input (50ms) (Input50)/Rear Left Radar(S0) Objects Information (RLRdr)/S0 Data Frame Read/Enabled Subsystem/M3ObjInfo/Subsystem1 ==
  const : Inport
  RemainderCnt : Inport  Port=2
  In : Inport  Port=3
  If : If  IfExpression=u1 >=0
  If Action Subsystem : Subsystem  TreatAsAtomicUnit=on
  If Action Subsystem1 : Subsystem  TreatAsAtomicUnit=on
  Merge : Merge
  Out : Outport
  wires:
  If Action Subsystem/1(Out1) -> Merge/1
  Merge/1 -> Out/1
  If/2 -> If Action Subsystem1/Action
  If Action Subsystem1/1(Out1) -> Merge/2
  If/1 -> If Action Subsystem/Action
  const/1 -> If/1
  In/1 -> If Action Subsystem1/1(In1)

== system DFADAS2_SenFus_v1_201204RC_training_210115/Signal Input (Input)/Signal Input (50ms) (Input50)/Rear Left Radar(S0) Objects Information (RLRdr)/S0 Data Frame Read/Enabled Subsystem/M4ObjInfo1/If Action Subsystem1 ==
  msg : Inport
  "MValueSel " : Inport  Port=2
  "obj_num " : Inport  Port=3
  Action Port : ActionPort  ActionType=then
  Add : Sum
  Add2 : Sum
  Gain : Gain  Gain=48
  MValueSel : Constant  Value=24
  MValueSel2 : Constant  Value=[1:24]
  Product : Product
  Scope3 : Scope
  Selector : Selector  InputPortWidth=240  IndexOptions=Index vector (port)  Indices=[1 3]  OutputSizes=1
  Selector1 : Selector  InputPortWidth=240  IndexOptions=Index vector (port)  Indices=[1 3]  OutputSizes=1
  M40ObjInfo : Outport
  M41ObjInfo : Outport  Port=2
  wires:
  "MValueSel "/1 -> Gain/1
  Gain/1 -> Add2/1
  msg/1 -> Selector1/1, Selector/1
  Add/1 -> Selector1/2
  MValueSel/1 -> Add/2
  Add2/1 -> Selector/2, Add/1
  MValueSel2/1 -> Add2/2
  Selector/1 -> M40ObjInfo/1
  Selector1/1 -> Product/1
  "obj_num "/1 -> Product/2, Scope3/1
  Product/1 -> M41ObjInfo/1

== system DFADAS2_SenFus_v1_201204RC_training_210115/Signal Input (Input)/Signal Input (50ms) (Input50)/Rear Left Radar(S0) Objects Information (RLRdr)/S0 Data Frame Read/Enabled Subsystem/M4ObjInfo1/If Action Subsystem2 ==
  Action Port : ActionPort  ActionType=elseif
  Constant : Constant  Value=[0 0 0 0 0 0 0 0 0 0 0 0 0 0 0 0 0 0 0 0 0 0 0 0]
  Constant1 : Constant  Value=[0 0 0 0 0 0 0 0 0 0 0 0 0 0 0 0 0 0 0 0 0 0 0 0]
  ZeroObjInfo0 : Outport
  ZeroObjInfo1 : Outport  Port=2
  wires:
  Constant/1 -> ZeroObjInfo0/1
  Constant1/1 -> ZeroObjInfo1/1

== system DFADAS2_SenFus_v1_201204RC_training_210115/Signal Input (Input)/Signal Input (50ms) (Input50)/Rear Left Radar(S0) Objects Information (RLRdr)/S0 Data Frame Read/Enabled Subsystem/M4ObjInfo1/Subsystem1 ==
  const : Inport
  RemainderCnt : Inport  Port=2
  In : Inport  Port=3
  If : If  IfExpression=u1 >=0
  If Action Subsystem : Subsystem  TreatAsAtomicUnit=on
  If Action Subsystem1 : Subsystem  TreatAsAtomicUnit=on
  Merge : Merge
  Out : Outport
  wires:
  If Action Subsystem/1(Out1) -> Merge/1
  Merge/1 -> Out/1
  If/2 -> If Action Subsystem1/Action
  If Action Subsystem1/1(Out1) -> Merge/2
  If/1 -> If Action Subsystem/Action
  const/1 -> If/1
  In/1 -> If Action Subsystem1/1(In1)

== system DFADAS2_SenFus_v1_201204RC_training_210115/Signal Input (Input)/Signal Input (50ms) (Input50)/Rear Left Radar(S0) Objects Information (RLRdr)/S0 Data Frame Read/Enabled Subsystem/Unpack/If Action Subsystem ==
  msg : Inport
  Action Port : ActionPort  ActionType=then
  Unpack : Subsystem
  RLRdrObjInfo : Outport
  MValue : Outport  Port=2
  wires:
  Unpack/2(MValue1) -> MValue/1
  msg/1 -> Unpack/1(msg)
  Unpack/1(RLRdrObjInfo1) -> RLRdrObjInfo/1

== system DFADAS2_SenFus_v1_201204RC_training_210115/Signal Input (Input)/Signal Input (50ms) (Input50)/Rear Left Radar(S0) Objects Information (RLRdr)/S0 Data Frame Read/Enabled Subsystem/Unpack/If Action Subsystem1 ==
  Action Port : ActionPort  ActionType=elseif
  Constant : Constant  Value=99
  DflMValue : Outport
  wires:
  Constant/1 -> DflMValue/1

== system DFADAS2_SenFus_v1_201204RC_training_210115/Signal Input (Input)/Signal Input (50ms) (Input50)/Rear Right Radar(S1) Objects Information (RRRdr)/S0 Data Frame Read/Enabled Subsystem/M0ObjInfo/If Action Subsystem1 ==
  msg : Inport
  "MValueSel " : Inport  Port=2
  obj_trufal : Inport  Port=3
  Action Port : ActionPort  ActionType=then
  Add : Sum
  Add2 : Sum
  MValueSel : Constant  Value=24
  MValueSel2 : Constant  Value=[1:24]
  Product : Product
  Scope1 : Scope
  Selector : Selector  InputPortWidth=240  IndexOptions=Index vector (port)  Indices=[1 3]  OutputSizes=1
  Selector1 : Selector  InputPortWidth=240  IndexOptions=Index vector (port)  Indices=[1 3]  OutputSizes=1
  M00ObjInfo : Outport
  M01ObjInfo : Outport  Port=2
  wires:
  Product/1 -> M01ObjInfo/1
  obj_trufal/1 -> Scope1/1, Product/2
  Selector1/1 -> Product/1
  Selector/1 -> M00ObjInfo/1
  "MValueSel "/1 -> Add2/1
  MValueSel2/1 -> Add2/2
  Add2/1 -> Add/1, Selector/2
  MValueSel/1 -> Add/2
  Add/1 -> Selector1/2
  msg/1 -> Selector1/1, Selector/1

== system DFADAS2_SenFus_v1_201204RC_training_210115/Signal Input (Input)/Signal Input (50ms) (Input50)/Rear Right Radar(S1) Objects Information (RRRdr)/S0 Data Frame Read/Enabled Subsystem/M0ObjInfo/If Action Subsystem2 ==
  Action Port : ActionPort  ActionType=elseif
  Constant : Constant  Value=[0 0 0 0 0 0 0 0 0 0 0 0 0 0 0 0 0 0 0 0 0 0 0 0]
  Constant1 : Constant  Value=[0 0 0 0 0 0 0 0 0 0 0 0 0 0 0 0 0 0 0 0 0 0 0 0]
  ZeroObjInfo0 : Outport
  ZeroObjInfo1 : Outport  Port=2
  wires:
  Constant1/1 -> ZeroObjInfo1/1
  Constant/1 -> ZeroObjInfo0/1

== system DFADAS2_SenFus_v1_201204RC_training_210115/Signal Input (Input)/Signal Input (50ms) (Input50)/Rear Right Radar(S1) Objects Information (RRRdr)/S0 Data Frame Read/Enabled Subsystem/M0ObjInfo/Subsystem1 ==
  const : Inport
  RemainderCnt : Inport  Port=2
  In : Inport  Port=3
  If : If  IfExpression=u1 >=0
  If Action Subsystem : Subsystem  TreatAsAtomicUnit=on
  If Action Subsystem1 : Subsystem  TreatAsAtomicUnit=on
  Merge : Merge
  Out : Outport
  wires:
  In/1 -> If Action Subsystem1/1(In1)
  const/1 -> If/1
  If/1 -> If Action Subsystem/Action
  If Action Subsystem1/1(Out1) -> Merge/2
  If/2 -> If Action Subsystem1/Action
  Merge/1 -> Out/1
  If Action Subsystem/1(Out1) -> Merge/1

== system DFADAS2_SenFus_v1_201204RC_training_210115/Signal Input (Input)/Signal Input (50ms) (Input50)/Rear Right Radar(S1) Objects Information (RRRdr)/S0 Data Frame Read/Enabled Subsystem/M1ObjInfo1/If Action Subsystem1 ==
  msg : Inport
  "MValueSel " : Inport  Port=2
  "0bj_d4 " : Inport  Port=3
  Action Port : ActionPort  ActionType=then
  Add : Sum
  Add2 : Sum
  Gain : Gain  Gain=48
  MValueSel : Constant  Value=24
  MValueSel2 : Constant  Value=[1:24]
  Product : Product
  Scope3 : Scope
  Selector : Selector  InputPortWidth=240  IndexOptions=Index vector (port)  Indices=[1 3]  OutputSizes=1
  Selector1 : Selector  InputPortWidth=240  IndexOptions=Index vector (port)  Indices=[1 3]  OutputSizes=1
  M10ObjInfo : Outport
  M11ObjInfo : Outport  Port=2
  wires:
  Selector/1 -> M10ObjInfo/1
  Product/1 -> M11ObjInfo/1
  "0bj_d4 "/1 -> Scope3/1, Product/2
  "MValueSel "/1 -> Gain/1
  Gain/1 -> Add2/1
  msg/1 -> Selector1/1, Selector/1
  Add/1 -> Selector1/2
  MValueSel/1 -> Add/2
  Add2/1 -> Selector/2, Add/1
  MValueSel2/1 -> Add2/2
  Selector1/1 -> Product/1

== system DFADAS2_SenFus_v1_201204RC_training_210115/Signal Input (Input)/Signal Input (50ms) (Input50)/Rear Right Radar(S1) Objects Information (RRRdr)/S0 Data Frame Read/Enabled Subsystem/M1ObjInfo1/If Action Subsystem2 ==
  Action Port : ActionPort  ActionType=elseif
  Constant : Constant  Value=[0 0 0 0 0 0 0 0 0 0 0 0 0 0 0 0 0 0 0 0 0 0 0 0]
  Constant1 : Constant  Value=[0 0 0 0 0 0 0 0 0 0 0 0 0 0 0 0 0 0 0 0 0 0 0 0]
  ZeroObjInfo0 : Outport
  ZeroObjInfo1 : Outport  Port=2
  wires:
  Constant/1 -> ZeroObjInfo0/1
  Constant1/1 -> ZeroObjInfo1/1

== system DFADAS2_SenFus_v1_201204RC_training_210115/Signal Input (Input)/Signal Input (50ms) (Input50)/Rear Right Radar(S1) Objects Information (RRRdr)/S0 Data Frame Read/Enabled Subsystem/M1ObjInfo1/Subsystem1 ==
  const : Inport
  RemainderCnt : Inport  Port=2
  In : Inport  Port=3
  If : If  IfExpression=u1 >=0
  If Action Subsystem : Subsystem  TreatAsAtomicUnit=on
  If Action Subsystem1 : Subsystem  TreatAsAtomicUnit=on
  Merge : Merge
  Out : Outport
  wires:
  In/1 -> If Action Subsystem1/1(In1)
  const/1 -> If/1
  If/1 -> If Action Subsystem/Action
  If Action Subsystem1/1(Out1) -> Merge/2
  If/2 -> If Action Subsystem1/Action
  Merge/1 -> Out/1
  If Action Subsystem/1(Out1) -> Merge/1

== system DFADAS2_SenFus_v1_201204RC_training_210115/Signal Input (Input)/Signal Input (50ms) (Input50)/Rear Right Radar(S1) Objects Information (RRRdr)/S0 Data Frame Read/Enabled Subsystem/M2ObjInfo/If Action Subsystem1 ==
  msg : Inport
  "MValueSel " : Inport  Port=2
  "obj_count_trorfa " : Inport  Port=3
  Action Port : ActionPort  ActionType=then
  Add : Sum
  Add2 : Sum
  Gain : Gain  Gain=48
  MValueSel : Constant  Value=24
  MValueSel2 : Constant  Value=[1:24]
  Product : Product
  Scope3 : Scope
  Selector : Selector  InputPortWidth=240  IndexOptions=Index vector (port)  Indices=[1 3]  OutputSizes=1
  Selector1 : Selector  InputPortWidth=240  IndexOptions=Index vector (port)  Indices=[1 3]  OutputSizes=1
  M20ObjInfo : Outport
  M21ObjInfo : Outport  Port=2
  wires:
  Product/1 -> M21ObjInfo/1
  "obj_count_trorfa "/1 -> Scope3/1, Product/2
  Selector1/1 -> Product/1
  Selector/1 -> M20ObjInfo/1
  MValueSel2/1 -> Add2/2
  Add2/1 -> Add/1, Selector/2
  MValueSel/1 -> Add/2
  Add/1 -> Selector1/2
  msg/1 -> Selector/1, Selector1/1
  Gain/1 -> Add2/1
  "MValueSel "/1 -> Gain/1

== system DFADAS2_SenFus_v1_201204RC_training_210115/Signal Input (Input)/Signal Input (50ms) (Input50)/Rear Right Radar(S1) Objects Information (RRRdr)/S0 Data Frame Read/Enabled Subsystem/M2ObjInfo/If Action Subsystem2 ==
  Action Port : ActionPort  ActionType=elseif
  Constant : Constant  Value=[0 0 0 0 0 0 0 0 0 0 0 0 0 0 0 0 0 0 0 0 0 0 0 0]
  Constant1 : Constant  Value=[0 0 0 0 0 0 0 0 0 0 0 0 0 0 0 0 0 0 0 0 0 0 0 0]
  ZeroObjInfo0 : Outport
  ZeroObjInfo1 : Outport  Port=2
  wires:
  Constant1/1 -> ZeroObjInfo1/1
  Constant/1 -> ZeroObjInfo0/1
